simulink model "CAD_test4_2"  (R2019a)
settings: Solver=VariableStepAuto  StartTime=0.0  StopTime=20.0  RelTol=1e-3
settings Model: Creator=83621  LastModifiedBy=83621

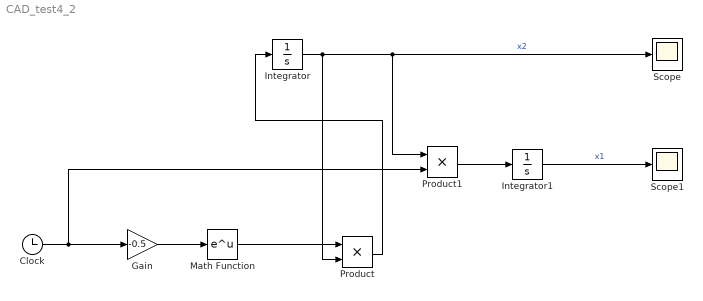
== system CAD_test4_2 ==
  Clock : Clock
  Gain : Gain  Gain=-0.5
  Integrator : Integrator  InitialCondition=1
  Integrator1 : Integrator  InitialCondition=1
  Math Function : Math  SaturateOnIntegerOverflow=on
  Product : Product
  Product1 : Product
  Scope : Scope
  Scope1 : Scope
  wires:
  Math Function/1 -> Product/1
  Clock/1 -> Product1/2, Gain/1
  Gain/1 -> Math Function/1
  Integrator/1 -> Scope/1, Product1/1, Product/2  "x2"
  Product/1 -> Integrator/1
  Product1/1 -> Integrator1/1
  Integrator1/1 -> Scope1/1  "x1"
